simulink model "sf phase 2 psd only"  (R2024b)
settings: Solver=VariableStepAuto  StartTime=0.0  StopTime=10.0  RelTol=1e-3
libraries: simulink x2, dspxfrm3 x2, dspsigops x2
settings Model: Creator=potat  LastModifiedBy=potat

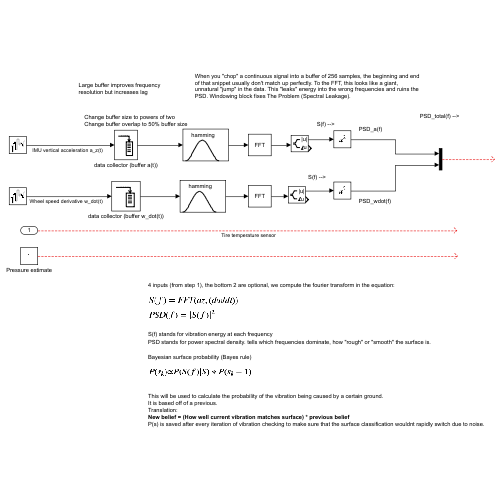
[thumbnail: Simulink's stored preview of the top-level diagram]
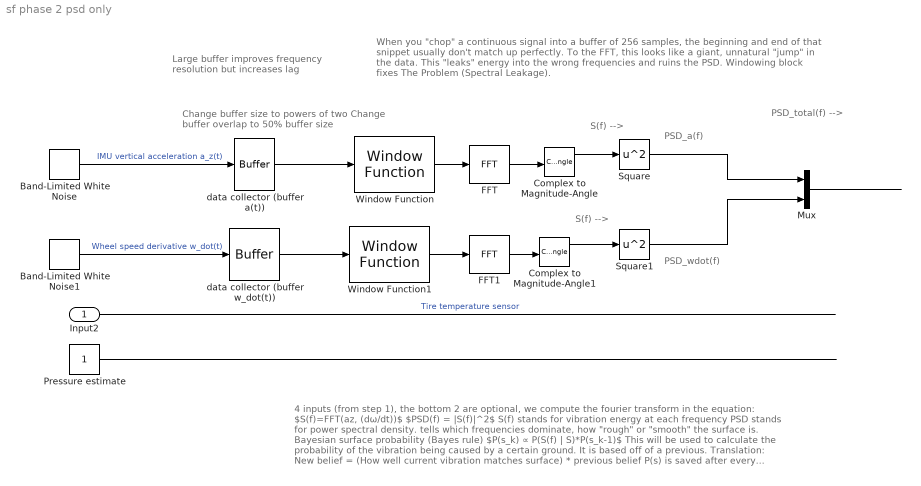
== system sf phase 2 psd only ==
  note: When you "chop" a continuous signal into a buffer of 256 samples, the beginning and end of that snippet usually don't match up perfectly. To the FFT, this looks like a giant, unnatural "jump" in the data. This "leaks" energy into the wrong frequencies and ruins the PSD. Windowing block fixes The Problem (Spectral Leakage).
  note: Large buffer improves frequency resolution but increases lag
  note: Change buffer size to powers of two
      | Change buffer overlap to 50% buffer size
  note: PSD_total(f) -->
  note: S(f) -->
  note: 4 inputs (from step 1), the bottom 2 are optional, we compute the fourier transform in the equation:
      |
      | $S(f)=FFT(az​, (dω/dt))$
      | $PSD(f) = |S(f)|^2$
      |
      | S(f) stands for vibration energy at each frequency
      | PSD stands for power spectral density. tells which frequencies dominate, how "rough" or "smooth" the surface is.
      |
      | Bayesian surface probability (Bayes rule)
      |
      | $P(s_k) ∝ P(S(f) | S)*P(s_k-1)$
      |
      | This will be used to calculate the probability of the vibration being caused by a certain ground.
      | It is based off of a previous.
      | Translation:
      | New belief = (How well current vibration matches surface) * previous belief
      | P(s) is saved after every iteration of vibration checking to make sure that the surface classification wouldnt rapidly switch due to noise.
  note: S(f) -->
  note: PSD_a(f)
  note: PSD_wdot(f)
  Input2 : Inport
  Band-Limited White Noise : simulink/Sources/Band-Limited White Noise  Cov=[0.1]  Ts=0.001  seed=[23341]
  Band-Limited White Noise1 : simulink/Sources/Band-Limited White Noise  Cov=[0.1]  Ts=0.001  seed=[23341]
  Complex to Magnitude-Angle : ComplexToMagnitudeAngle
  Complex to Magnitude-Angle1 : ComplexToMagnitudeAngle
  FFT : dspxfrm3/FFT  FFTImplementation=Auto  CompMethod=Table lookup  TableOpt=NEW  TableOptActive=Speed  BitRevOrder=off  Normalize=off  InheritFFTLength=on  FFTLength=64  WrapInput=on  roundingMode=Ceiling  overflowMode=off  firstCoeffDataTypeStr=Inherit: Same word length as input  firstCoeffLastDataTypeStr=Inherit: Same word length as input  outputMin=[]  outputMax=[]
  FFT1 : dspxfrm3/FFT  FFTImplementation=Auto  CompMethod=Table lookup  TableOpt=NEW  TableOptActive=Speed  BitRevOrder=off  Normalize=off  InheritFFTLength=on  FFTLength=64  WrapInput=on  roundingMode=Ceiling  overflowMode=off  firstCoeffDataTypeStr=Inherit: Same word length as input  firstCoeffLastDataTypeStr=Inherit: Same word length as input  outputMin=[]  outputMax=[]
  Mux : Mux  Inputs=2
  Pressure estimate : Constant
  Square : Math  Operator=square
  Square1 : Math  Operator=square
  Window Function : dspsigops/Window Function  winmode=Apply window to input  wintype=Hamming  sampmode=Continuous  samptime=1  N=64  Rs=50  beta=10  winsamp=Symmetric  UserWindow=hamming  OptParams=off  UserParams={'symmetric'}  dataType=double  isSigned=on  wordLen=16  udDataType=sfix(16)  fracBitsMode=Best precision  numFracBits=15  roundingMode=Floor  overflowMode=off  numSidelobes=4  sidelobeLevel=-30
  Window Function1 : dspsigops/Window Function  winmode=Apply window to input  wintype=Hamming  sampmode=Continuous  samptime=1  N=64  Rs=50  beta=10  winsamp=Symmetric  UserWindow=hamming  OptParams=off  UserParams={'symmetric'}  dataType=double  isSigned=on  wordLen=16  udDataType=sfix(16)  fracBitsMode=Best precision  numFracBits=15  roundingMode=Floor  overflowMode=off  numSidelobes=4  sidelobeLevel=-30
  data collector (buffer a(t)) : Buffer  N=128  V=64  OutputFrames=off
  data collector (buffer w_dot(t)) : Buffer  N=128  V=64  OutputFrames=off
  wires:
  Band-Limited White Noise/1 -> data collector (buffer a(t))/1  "IMU vertical acceleration a_z(t)"
  Band-Limited White Noise1/1 -> data collector (buffer w_dot(t))/1  "Wheel speed derivative w_dot(t)"
  Input2/1 -> ?  "Tire temperature sensor"
  Pressure estimate/1 -> ?
  FFT/1 -> Complex to Magnitude-Angle/1
  data collector (buffer a(t))/1 -> Window Function/1
  Complex to Magnitude-Angle/1 -> Square/1
  data collector (buffer w_dot(t))/1 -> Window Function1/1
  FFT1/1 -> Complex to Magnitude-Angle1/1
  Complex to Magnitude-Angle1/1 -> Square1/1
  Square/1 -> Mux/1
  Window Function/1 -> FFT/1
  Window Function1/1 -> FFT1/1
  Square1/1 -> Mux/2
  Mux/1 -> ?
